simulink model "az10"  (R2016b)
settings: Solver=VariableStepAuto  StartTime=0.0  StopTime=10.0  RelTol=1e-3
libraries: fuzblock x1
settings Model: Creator=Yasna  LastModifiedBy=Yasna

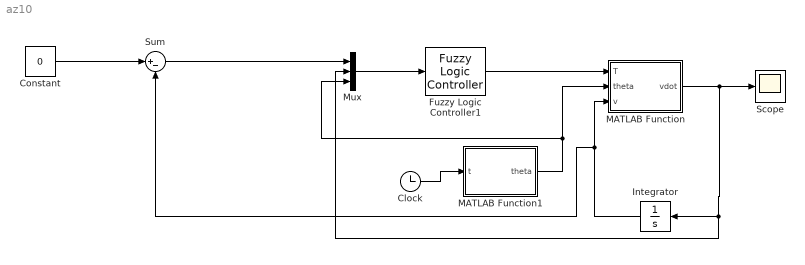
== system az10 ==
  Clock : Clock
  Constant : Constant  Value=0
  Fuzzy Logic Controller1 : fuzblock/Fuzzy Logic  Controller  fis='vehicle.fis'
  Integrator : Integrator
  MATLAB Function : MATLAB Function  TreatAsAtomicUnit=on
  MATLAB Function1 : MATLAB Function  TreatAsAtomicUnit=on
  Mux : Mux  Inputs=3
  Scope : Scope
  Sum : Sum  Inputs=|+-
  wires:
  Integrator/1 -> Sum/2, MATLAB Function/3(v)
  Fuzzy Logic Controller1/1 -> MATLAB Function/1(T)
  Constant/1 -> Sum/1
  Sum/1 -> Mux/1
  Mux/1 -> Fuzzy Logic Controller1/1
  MATLAB Function/1(vdot) -> Scope/1, Mux/2, Integrator/1
  Clock/1 -> MATLAB Function1/1(t)
  MATLAB Function1/1(theta) -> MATLAB Function/2(theta), Mux/3

== matlab function az10/MATLAB Function1 ==
  data: t input; theta output
function theta = fcn(t)
theta=0;
if t>0
if t<20
theta=(0.25*t)-5;
elseif t<40
theta=0;
elseif t<80
theta=(0.25*t)-10;
elseif t<100
theta=10;
end
end

== matlab function az10/MATLAB Function ==
  data: T input; vdot output; theta input; v input
function vdot = fcn(T,theta,v)
vdot=-0.1*v-T+0.1*theta;
